simulink model "matrixconcatenation_tut1"  (Simulink 5.0)
settings: Solver=FixedStepDiscrete  StartTime=0.0  StopTime=10.0  RelTol=1e-3
PreLoadFcn:
  | dsp_examples_A = [1:10;1 1 0 0 1 1 0 0 1 1]';
PostLoadFcn:
  | set_param(gcs,'SimulationCommand','Update')
libraries: dspsrcs4 x4, simulink x2
settings Model: RequirementInfo=9  Creator=ckamachi  LastModifiedBy=ckamachi  ExtModeTrigMode=oneshot  ExtModeArmWhenConnect=off  LimitDataPoints=off  BlockReductionOpt=off  BooleanDataType=off

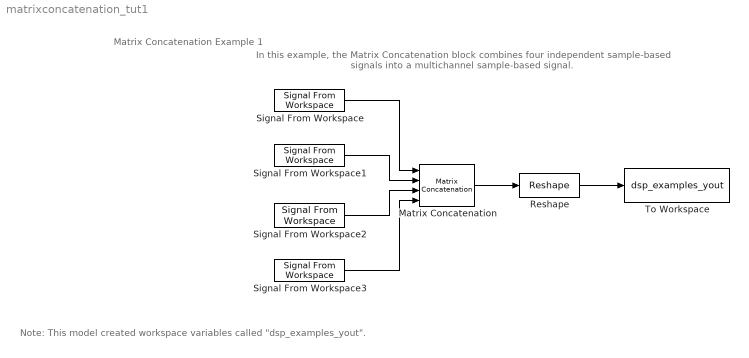
== system matrixconcatenation_tut1 ==
  note: Matrix Concatenation Example 1
  note: In this example, the Matrix Concatenation block combines
      | four independent sample-based signals into a multichannel
      | sample-based signal.
  note: Note: This model created workspace variables called "dsp_examples_yout".
  Matrix Concatenation : simulink/Math Operations/Matrix Concatenation  numInports=4  catMethod=Vertical
  Reshape : simulink/Math Operations/Reshape  OutputDimensionality=Customize  OutputDimensions=[2,2]
  Signal From Workspace : dspsrcs4/Signal From Workspace  X=1:10  Ts=1  nsamps=1  OutputAfterFinalValue=Setting to zero
  Signal From Workspace1 : dspsrcs4/Signal From Workspace  X=-1:-1:-10  Ts=1  nsamps=1  OutputAfterFinalValue=Setting to zero
  Signal From Workspace2 : dspsrcs4/Signal From Workspace  X=zeros(10,1)  Ts=1  nsamps=1  OutputAfterFinalValue=Setting to zero
  Signal From Workspace3 : dspsrcs4/Signal From Workspace  X=5*ones(10,1)  Ts=1  nsamps=1  OutputAfterFinalValue=Setting to zero
  To Workspace : ToWorkspace  VariableName=dsp_examples_yout  SampleTime=-1  SaveFormat=Array
  wires:
  Signal From Workspace/1 -> Matrix Concatenation/1
  Signal From Workspace3/1 -> Matrix Concatenation/4
  Signal From Workspace1/1 -> Matrix Concatenation/2
  Signal From Workspace2/1 -> Matrix Concatenation/3
  Reshape/1 -> To Workspace/1
  Matrix Concatenation/1 -> Reshape/1
